simulink model "speed_controller_load"  (R2022a)
settings: Solver=VariableStepAuto  StartTime=0.0  StopTime=180  RelTol=1e-3
values from neighbouring files (symbols this model uses):
  B = 0.0000464    (= 4.64e-05)    [simConstants.m]
  J = 0.0000109    (= 1.09e-05)    [simConstants.m]
  k_e = 0.0348    [simConstants.m]
  k_t = 0.0348    [simConstants.m]
  L = 0.00042    [simConstants.m]
  R_a = 4.89    [simConstants.m]
libraries: cstblocks x1
settings Model: Creator=nickk  LastModifiedBy=nickk

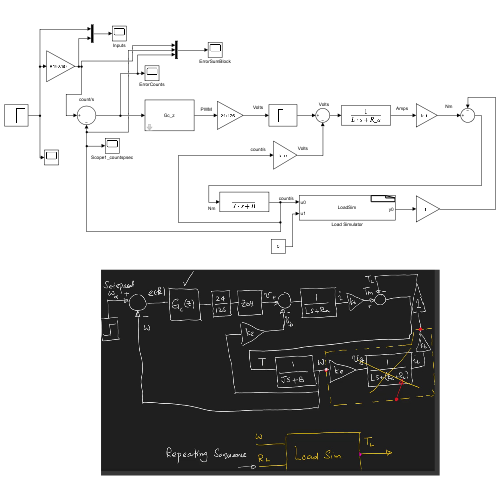
[thumbnail: Simulink's stored preview of the top-level diagram]
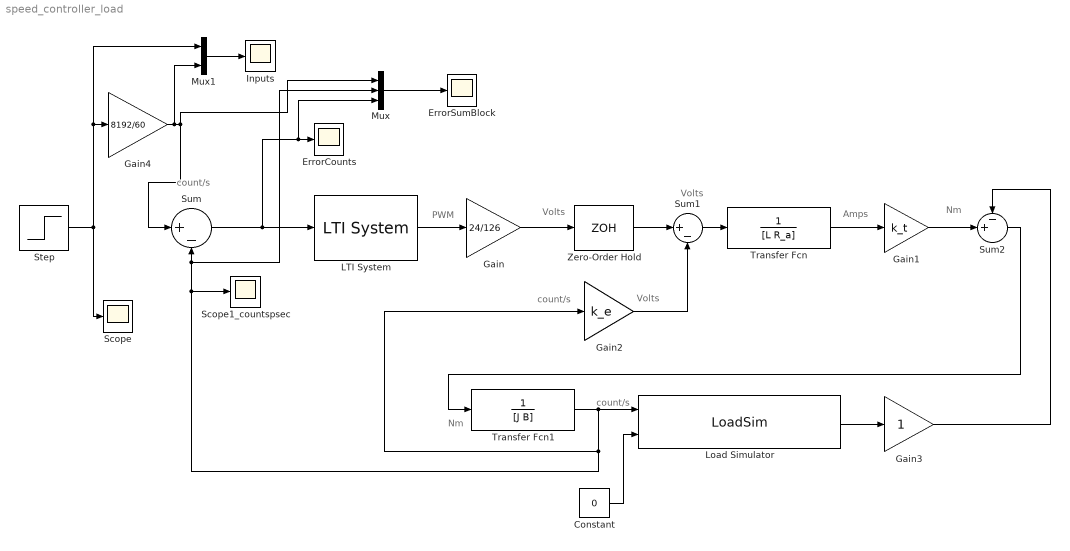
== system speed_controller_load ==
  note: Nm
  note: Amps
  note: Volts
  note: PWM
  note: count/s
  note: Nm
  note: Volts
  note: count/s
  note: Volts
  note: count/s
  Constant : Constant  Value=0
  ErrorCounts : Scope
  ErrorSumBlock : Scope
  Gain : Gain  Gain=24/126
  Gain1 : Gain  Gain=k_t
  Gain2 : Gain  Gain=k_e
  Gain3 : Gain
  Gain4 : Gain  Gain=8192/60
  Inputs : Scope
  LTI System : cstblocks/LTI System  sys=Gc_z  IC=[]
  "Load Simulator " : S-Function  InitFcn=try, set_param(gcb,'FunctionName','LoadSim'), end  FunctionName=LoadSim  SFunctionModules=LoadSim_wrapper  SFunctionDeploymentMode=off  EnableBusSupport=off  mask(S-Function Builder){}
      mask help: Simulink:masks:SFunctionBuilder_MD
      mask init:
      | val = [[.9  0.75 0.75 1 1 .9 .9 1]',[1 1 0.75 0.75 .9 .9 1 .9]'];try , sys = get_param(gcb,'SfunBuilderFcnName');if isempty(sys), sys = get_param(gcb,'FunctionName'); end,catch, sys = get_param(gcb,'FunctionName'); end
      settings: CopyFcn=set_param(gcbh,'LinkStatus','none')  PreSaveFcn=try, set_param(gcb,'FunctionName','LoadSim'), end  OpenFcn=sfunctionwizard(gcbh)
      mask Display:
      | plot(val(:,1),val(:,2))
      | disp(sys)
      | port_label('input',1,'u0')
      | port_label('input',2,'u1')
      | port_label('output',1,'y0')
  Mux : Mux  Inputs=3
  Mux1 : Mux  Inputs=2
  Scope : Scope
  Scope1_countspsec : Scope
  Step : Step  Time=15  Before=1000  After=2000  SampleTime=0
  Sum : Sum  Inputs=|+-
  Sum1 : Sum  Inputs=|+-
  Sum2 : Sum  Inputs=-+|
  Transfer Fcn : TransferFcn  Denominator=[L R_a]
  Transfer Fcn1 : TransferFcn  Denominator=[J B]
  Zero-Order Hold : ZeroOrderHold  SampleTime=-1
  wires:
  Gain/1 -> Zero-Order Hold/1
  Zero-Order Hold/1 -> Sum1/1
  Gain1/1 -> Sum2/2
  Gain2/1 -> Sum1/2
  "Load Simulator "/1 -> Gain3/1
  Gain3/1 -> Sum2/1
  LTI System/1 -> Gain/1
  Sum/1 -> Mux/3, ErrorCounts/1, LTI System/1
  Sum1/1 -> Transfer Fcn/1
  Transfer Fcn/1 -> Gain1/1
  Transfer Fcn1/1 -> Gain2/1, Mux/2, Sum/2, Scope1_countspsec/1, "Load Simulator "/1
  Constant/1 -> "Load Simulator "/2
  Sum2/1 -> Transfer Fcn1/1
  Step/1 -> Scope/1, Mux1/1, Gain4/1
  Gain4/1 -> Mux1/2, Mux/1, Sum/1
  Mux1/1 -> Inputs/1
  Mux/1 -> ErrorSumBlock/1
